simulink model "Simple_Cruise_cf"  (R2014b)
settings: Solver=ode45  StartTime=0.0  StopTime=180  RelTol=1e-3
InitFcn:
  | m=1000;
  | b=50;
  | u=500;
StopFcn:
  | plot(v)
  | grid
settings Model: Creator=Administrator  LastModifiedBy=Administrator

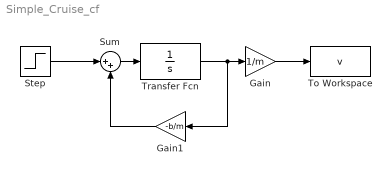
== system Simple_Cruise_cf ==
  Gain : Gain  Gain=1/m
  Gain1 : Gain  Gain=-b/m
  Step : Step  Time=0  Before=500  After=500  SampleTime=0.01
  Sum : Sum  Inputs=|++
  To Workspace : ToWorkspace  VariableName=v  SaveFormat=Timeseries  SampleTime=-1
  Transfer Fcn : TransferFcn  Denominator=[1 0]
  wires:
  Step/1 -> Sum/1
  Sum/1 -> Transfer Fcn/1
  Gain1/1 -> Sum/2
  Transfer Fcn/1 -> Gain1/1, Gain/1
  Gain/1 -> To Workspace/1
